simulink model "lqr_model"  (R2024a)
settings: Solver=FixedStepAuto  StartTime=0.0  StopTime=3  FixedStep=0.0001  MinStep=1e-8  RelTol=1e-8  AbsTol=1e-8
model workspace (MAT data in the model file):
  A = [11  -2  13; 6  -1  6; -6  -1  -8]
  B = [2; 0; 0]
  K = [-4 2.4167 -3]
values from neighbouring files (symbols this model uses):
  K1 = -inv(R1)*B'*P1    [lqr.m]
  K2 = -inv(R2)*B'*P2    [lqr.m]
  K3 = -inv(R3)*B'*P3    [lqr.m]
  K4 = -inv(R4)*B'*P4    [lqr.m]
settings Model: Creator=ventus  LastModifiedBy=ventus

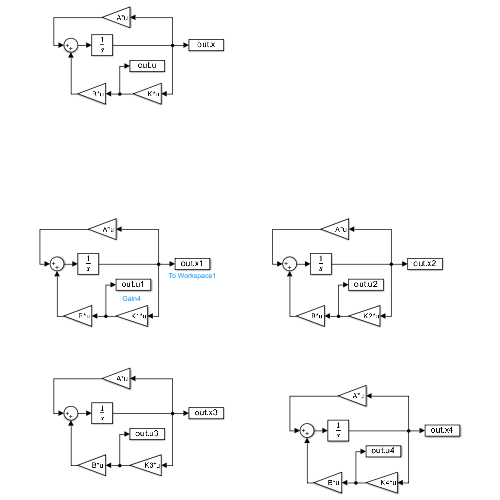
[thumbnail: Simulink's stored preview of the top-level diagram]
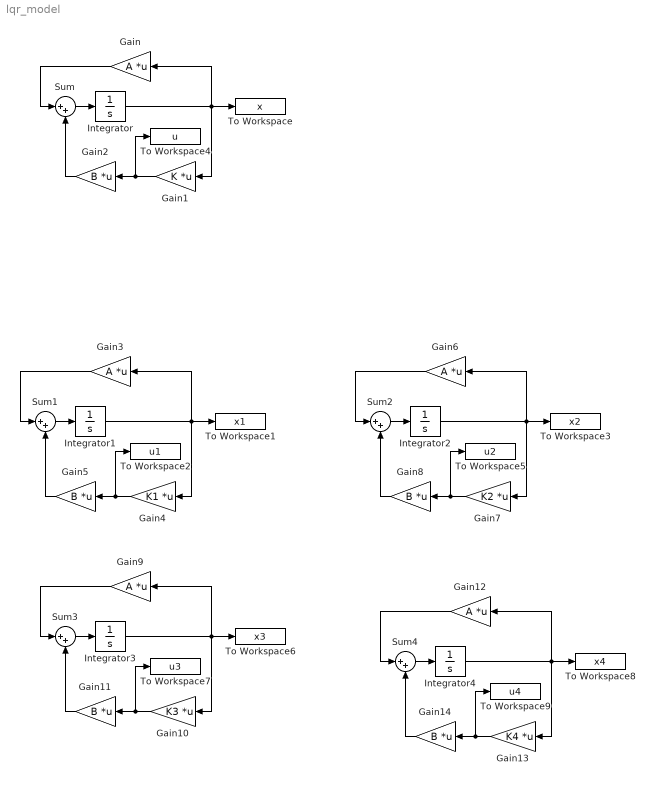
== system lqr_model ==
  Gain{,3,6,9,12} (5 alike) : Gain  Gain=A  Multiplication=Matrix(K*u)
  Gain1 : Gain  Gain=K  Multiplication=Matrix(K*u)
  Gain10 : Gain  Gain=K3  Multiplication=Matrix(K*u)
  Gain{2,5,8,11,14} (5 alike) : Gain  Gain=B  Multiplication=Matrix(K*u)
  Gain13 : Gain  Gain=K4  Multiplication=Matrix(K*u)
  Gain4 : Gain  Gain=K1  Multiplication=Matrix(K*u)
  Gain7 : Gain  Gain=K2  Multiplication=Matrix(K*u)
  Integrator{,1..4} (5 alike) : Integrator  InitialCondition=[1; 1; 1]
  Sum{,1..4} (5 alike) : Sum  Inputs=|++
  To Workspace : ToWorkspace  VariableName=x  SaveFormat=Timeseries  SampleTime=-1
  To Workspace1 : ToWorkspace  VariableName=x1  SaveFormat=Timeseries  SampleTime=-1
  To Workspace2 : ToWorkspace  VariableName=u1  SaveFormat=Timeseries  SampleTime=-1
  To Workspace3 : ToWorkspace  VariableName=x2  SaveFormat=Timeseries  SampleTime=-1
  To Workspace4 : ToWorkspace  VariableName=u  SaveFormat=Timeseries  SampleTime=-1
  To Workspace5 : ToWorkspace  VariableName=u2  SaveFormat=Timeseries  SampleTime=-1
  To Workspace6 : ToWorkspace  VariableName=x3  SaveFormat=Timeseries  SampleTime=-1
  To Workspace7 : ToWorkspace  VariableName=u3  SaveFormat=Timeseries  SampleTime=-1
  To Workspace8 : ToWorkspace  VariableName=x4  SaveFormat=Timeseries  SampleTime=-1
  To Workspace9 : ToWorkspace  VariableName=u4  SaveFormat=Timeseries  SampleTime=-1
  wires:
  Integrator/1 -> Gain/1, To Workspace/1, Gain1/1
  Sum/1 -> Integrator/1
  Gain/1 -> Sum/1
  Gain1/1 -> Gain2/1, To Workspace4/1
  Gain2/1 -> Sum/2
  Gain5/1 -> Sum1/2
  Integrator1/1 -> Gain3/1, To Workspace1/1, Gain4/1
  Gain4/1 -> To Workspace2/1, Gain5/1
  Sum1/1 -> Integrator1/1
  Gain3/1 -> Sum1/1
  Gain8/1 -> Sum2/2
  Integrator2/1 -> Gain6/1, To Workspace3/1, Gain7/1
  Gain7/1 -> To Workspace5/1, Gain8/1
  Sum2/1 -> Integrator2/1
  Gain6/1 -> Sum2/1
  Gain11/1 -> Sum3/2
  Integrator3/1 -> Gain9/1, To Workspace6/1, Gain10/1
  Gain10/1 -> To Workspace7/1, Gain11/1
  Sum3/1 -> Integrator3/1
  Gain9/1 -> Sum3/1
  Gain14/1 -> Sum4/2
  Integrator4/1 -> Gain12/1, To Workspace8/1, Gain13/1
  Gain13/1 -> To Workspace9/1, Gain14/1
  Sum4/1 -> Integrator4/1
  Gain12/1 -> Sum4/1
